simulink model "impuls"  (Simulink 7.6)
settings: Solver=ode45  StartTime=0.0  StopTime=10000  RelTol=1e-3
values from neighbouring files (symbols this model uses):
  T = 800    [koef.m]
settings Model: Creator=Johannes  LastModifiedBy=Johannes  ExtModeTrigMode=oneshot  ExtModeArmWhenConnect=off
settings DataIOCC: LimitDataPoints=off
settings OptimizationCC: BlockReduction=off  BooleanDataType=off
settings DebuggingCC: SaveWithParameterizedLinksMsg=none  SignalResolutionControl=TryResolveAllWithWarning  SolverPrmCheckMsg=none  MultiTaskDSMMsg=warning  MultiTaskCondExecSysMsg=none  StrictBusMsg=None
settings HardwareCC: TargetUnknown=on
settings RTWCC: IncludeERTFirstTime=on

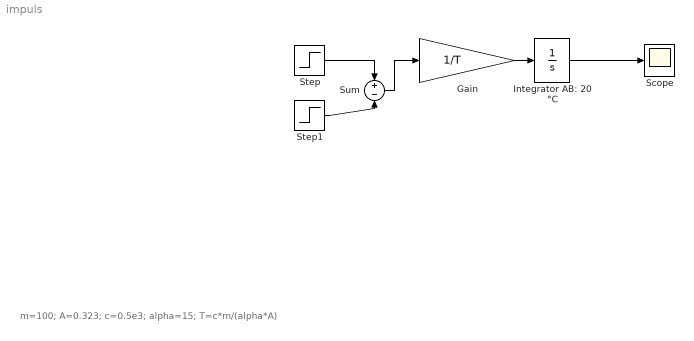
== system impuls ==
  note: m=100;
      | A=0.323;
      | c=0.5e3;
      | alpha=15;
      | T=c*m/(alpha*A)
  Gain : Gain  Gain=1/T  SaturateOnIntegerOverflow=on  OutDataTypeStr=Inherit: Same as input  ParamDataTypeStr=Inherit: Same as input
  Integrator AB: 20 °C : Integrator
  Scope : Scope
  Step : Step  Time=0  SampleTime=0
  Step1 : Step  Time=0.1  SampleTime=0
  Sum : Sum  Inputs=+-
  wires:
  Gain/1 -> Integrator AB: 20 °C/1
  Integrator AB: 20 °C/1 -> Scope/1
  Step1/1 -> Sum/2
  Step/1 -> Sum/1
  Sum/1 -> Gain/1
